simulink model "DualMotor_FaultTolerant_TorqueControl"  (R2025a)
settings: Solver=ode3  StartTime=0.0  StopTime=2  FixedStep=1e-6  RelTol=1e-3
libraries: spsDCVoltageSourceLib x2, spsGroundLib x2, eePmsmFieldOrientedControl x2, spsPermanentMagnetSynchronousMachineLib x2, spsUniversalBridgeLib x2, slpidlib x1, simulink x1, sps_lib x1
settings Model: Creator=lmh  LastModifiedBy=lmh

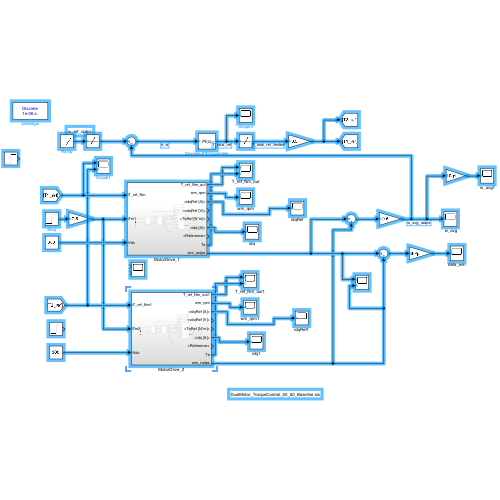
[thumbnail: Simulink's stored preview of the top-level diagram]
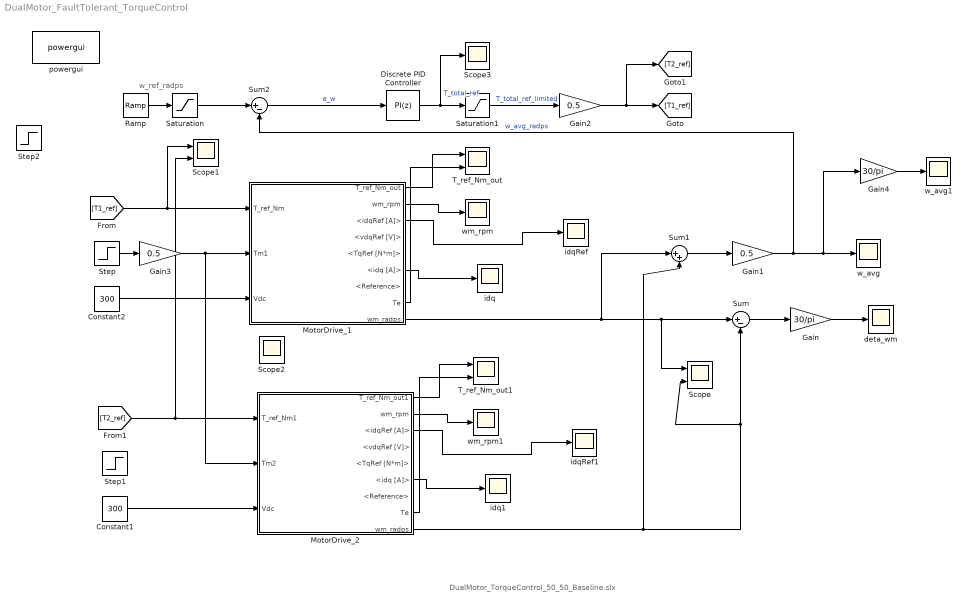
== system DualMotor_FaultTolerant_TorqueControl ==
  note: DualMotor_TorqueControl_50_50_Baseline.slx
  note: w_ref_radps
  " w_avg" : Scope
      settings: ActiveDisplayYMinimum=-1  ActiveDisplayYMaximum=1  DataLoggingVariableName=ScopeData10
  " w_avg1" : Scope
      settings: ActiveDisplayYMinimum=-42.23010556786226  ActiveDisplayYMaximum=380.07095011076035  DataLoggingVariableName=ScopeData11
  Constant1 : Constant  Value=300
  Constant2 : Constant  Value=300
  Discrete PID Controller : slpidlib/PID Controller  Controller=PI  Form=Parallel  TimeDomain=Discrete-time  UseExternalTs=off  SampleTime=1e-3  IntegratorMethod=Forward Euler  FilterMethod=Forward Euler  ControllerParametersSource=internal  P=0.2  I=0.3  UseKiTs=off  D=0  UseExternalDerivativeSource=off  N=100  UseFilter=on  TunerSelectOption=Transfer Function Based (PID Tuner App)  InitialConditionSource=internal  InitialConditionForIntegrator=0  InitialConditionForFilter=0  DifferentiatorICPrevScaledInput=0  ExternalReset=none  TrackingMode=off  Kt=1  LimitOutput=off  SatLimitsSource=internal  UpperSaturationLimit=inf  LowerSaturationLimit=-inf  LinearizeAsGain=off  AntiWindupMode=none  Kb=1  LimitIntegrator=off  UpperIntegratorSaturationLimit=inf  LowerIntegratorSaturationLimit=-inf  POutMin=[]  POutMax=[]  IOutMin=[]  IOutMax=[]  DOutMin=[]  DOutMax=[]  NOutMin=[]  NOutMax=[]  SumOutMin=[]  SumOutMax=[]  SaturationOutMin=[]  SaturationOutMax=[]  PParamMin=[]  PParamMax=[]  IParamMin=[]  IParamMax=[]  DParamMin=[]  DParamMax=[]  NParamMin=[]  NParamMax=[]  KbParamMin=[]  KbParamMax=[]  KtParamMin=[]  KtParamMax=[]  KbOutMin=[]  KbOutMax=[]  KtOutMin=[]  KtOutMax=[]  IntegratorOutMin=[]  IntegratorOutMax=[]  FilterOutMin=[]  FilterOutMax=[]  SumI1OutMin=[]  SumI1OutMax=[]  SumI2OutMin=[]  SumI2OutMax=[]  SumI3OutMin=[]  SumI3OutMax=[]  SumI4OutMin=[]  SumI4OutMax=[]  SumDOutMin=[]  SumDOutMax=[]  DifferentiatorOutMin=[]  DifferentiatorOutMax=[]  FilterDiffOutCoefMin=[]  FilterDiffOutCoefMax=[]  ReciprocalOutMin=[]  ReciprocalOutMax=[]  SumDenOutMin=[]  SumDenOutMax=[]  SumNumOutMin=[]  SumNumOutMax=[]  DivideOutMin=[]  DivideOutMax=[]  UdiffTsProdOutMin=[]  UdiffTsProdOutMax=[]  NTsProdOutMin=[]  NTsProdOutMax=[]  UintegralTsProdOutMin=[]  UintegralTsProdOutMax=[]  UngainTsProdOutMin=[]  UngainTsProdOutMax=[]  ClampingZeroOutDataTypeStr=Inherit: Inherit via back propagation  ClampingZeroOutMin=[]  ClampingZeroOutMax=[]  FilterDenConstantOutDataTypeStr=Inherit: Inherit via back propagation  FilterDenConstantOutMin=[]  FilterDenConstantOutMax=[]  PCopyOutDataTypeStr=Inherit: Inherit via back propagation  PCopyOutMin=[]  PCopyOutMax=[]  NCopyOutDataTypeStr=Inherit: Inherit via back propagation  NCopyOutMin=[]  NCopyOutMax=[]  IntegratorContinuousStateAttributes=''  IntegratorStateMustResolveToSignalObject=off  IntegratorRTWStateStorageClass=Auto  FilterContinuousStateAttributes=''  FilterStateMustResolveToSignalObject=off  FilterRTWStateStorageClass=Auto  ParallelPVariant=InternalParameters  IdealPVariant=Disabled  IVariant=InternalParameters  DVariant=Disabled  IntegratorVariant=Discrete  SatVariant=Disabled  AWVariant=Passthrough  PCopyVariant=Disabled  TRVariant=Disabled  FdbkBlocksVariant=Forward  IdealPFdbkVariant=Disabled  SatFdbkVariant=Disabled  DerivativeFilterVariant=Disabled  NVariant=Disabled  NCopyVariant=Disabled_SignalSpec  FilterICVariant=Disabled  IntegratorICVariant=InternalICs  ExternalResetVariant=Disabled  TRSumVariant=Passthrough  SumFdbkVariant=Disabled  SumVariant=Sum_PI  TsampFilterVariant=InternalTs  TsampNgainVariant=Passthrough  TsampIntegralVariant=Disabled_SignalSpec  ExternalSaturationOutDataTypeStr=Inherit: Same as second input  DerivativeSourceVariant=Disabled  PreIntVariant=InternalPreInt
      settings: LibrarySourceBlock=simulink/Discrete/Discrete PID Controller
  Gain : Gain  Gain=30/pi
  Gain1 : Gain  Gain=0.5
  Gain2 : Gain  Gain=0.5
  Gain3 : Gain  Gain=0.5
  Gain4 : Gain  Gain=30/pi
  MotorDrive_1 : Subsystem
  MotorDrive_2 : Subsystem
  Ramp : simulink/Sources/Ramp  slope=157.08  start=0.05  InitialOutput=0
  Saturation : Saturate  UpperLimit=31.416  LowerLimit=0
  Saturation1 : Saturate  UpperLimit=5  LowerLimit=-5
  Scope : Scope  NumInputPorts=2
      settings: ActiveDisplayYMinimum=-1  ActiveDisplayYMaximum=1  DataLoggingVariableName=ScopeData8
  Scope1 : Scope  NumInputPorts=2
      settings: ActiveDisplayYMinimum=-0.50042285131163777  ActiveDisplayYMaximum=0.992672654307302  DataLoggingVariableName=ScopeData12
  Scope2 : Scope  NumInputPorts=2
      settings: ActiveDisplayYMinimum=-0.40590531924916307  ActiveDisplayYMaximum=0.73013794484412364  DataLoggingVariableName=ScopeData13
  Scope3 : Scope
      settings: ActiveDisplayYMinimum=-0.97217317064289754  ActiveDisplayYMaximum=1.8423869448952914  DataLoggingVariableName=ScopeData14
  Step : Step  Time=0.3  SampleTime=1e-6
  Step1 : Step  Time=0.2  After=0.5  SampleTime=1e-6
  Step2 : Step  Time=0.2  After=0.5  SampleTime=1e-6
  Sum : Sum  Inputs=|+-
  Sum1 : Sum  Inputs=|++
  Sum2 : Sum  Inputs=|+-
  T_ref_Nm_out : Scope  NumInputPorts=2
      settings: ActiveDisplayYMinimum=-0.56957171237379067  ActiveDisplayYMaximum=1.0003558610919856
  T_ref_Nm_out1 : Scope  NumInputPorts=2
      settings: ActiveDisplayYMinimum=-1  ActiveDisplayYMaximum=1  DataLoggingVariableName=ScopeData6
  deta_wm : Scope
      settings: ActiveDisplayYMinimum=-1  ActiveDisplayYMaximum=1  DataLoggingVariableName=ScopeData9
  idq : Scope
      settings: ActiveDisplayYMinimum=-1.0831890867819363  ActiveDisplayYMaximum=1.2350252871725016  DataLoggingVariableName=ScopeData3
  idq1 : Scope
      settings: ActiveDisplayYMinimum=-0.803012654998282  ActiveDisplayYMaximum=1.1347435588564942  DataLoggingVariableName=ScopeData4
  idqRef : Scope
      settings: ActiveDisplayYMinimum=-0.26041666666666663  ActiveDisplayYMaximum=2.34375  DataLoggingVariableName=ScopeData2
  idqRef1 : Scope
      settings: ActiveDisplayYMinimum=-3.1835545787556114  ActiveDisplayYMaximum=2.3621352619007454  DataLoggingVariableName=ScopeData5
  powergui : sps_lib/powergui  Priority=1  SimulationMode=Discrete  SampleTime=1e-6  frequency=60  Iterations=50  frequencyindice=0  Pbase=100e6  ErrMax=1e-4  UnitsV=kV  UnitsW=MW  buscounter=0  FunctionMessages=off  echomessages=off  EnableUseOfTLC=off  CurrentSourceSwitches=off  DisableSnubberDevices=off  DisableRonSwitches=off  DisableVfSwitches=off  DisplayEquations=off  AutomaticDiscreteSolvers=off  SolverType=Tustin/Backward Euler (TBE)  Interpol=off  ExternalGateDelay=off  methode=off  Ts=100  x0status=blocks  SPID=on  SwTol=0  HookPort=off  NonlinearTolerance=1e-4  nMaxIteration=100  ContinueOnMaxIteration=off  RestoreLinks=warning  ResistiveCurrentMeasurement=off  Frange=[0:2:500]  Ylog=off  Xlog=on  ShowGrid=off  save=off  variable=ZData  structure=0  ZoomFFT=off  StartTime=0.0  cycles=1  DisplayStyle=1  fundamental=60  FreqAxis=off  MaxFrequency=1000  frequencyindicesteady=1  RmsSteady=1  display=off
  wm_rpm : Scope
      settings: ActiveDisplayYMinimum=-388.34435285098448  ActiveDisplayYMaximum=3465.7589265847746
  wm_rpm1 : Scope
      settings: ActiveDisplayYMinimum=-604.84980727002824  ActiveDisplayYMaximum=1187.9663788618518  DataLoggingVariableName=ScopeData7
  wires:
  Ramp/1 -> Saturation/1
  Sum/1 -> Gain/1
  MotorDrive_1/9(wm_radps) -> Sum1/1, Scope/1, Sum/1
  MotorDrive_2/3(<idqRef [A]>) -> idqRef1/1
  Step/1 -> Gain3/1
  MotorDrive_2/9(wm_radps) -> Scope/2, Sum/2, Sum1/2
  MotorDrive_2/1(T_ref_Nm_out1) -> T_ref_Nm_out1/1
  MotorDrive_2/2(wm_rpm) -> wm_rpm1/1
  Gain/1 -> deta_wm/1
  Constant2/1 -> MotorDrive_1/3(Vdc)
  MotorDrive_1/2(wm_rpm) -> wm_rpm/1
  Constant1/1 -> MotorDrive_2/3(Vdc)
  MotorDrive_1/1(T_ref_Nm_out) -> T_ref_Nm_out/1
  MotorDrive_1/6(<idq [A]>) -> idq/1
  MotorDrive_1/3(<idqRef [A]>) -> idqRef/1
  MotorDrive_2/6(<idq [A]>) -> idq1/1
  MotorDrive_1/8(Te) -> T_ref_Nm_out/2
  MotorDrive_2/8(Te) -> T_ref_Nm_out1/2
  Sum1/1 -> Gain1/1
  Gain1/1 -> Gain4/1, " w_avg"/1, Sum2/2  "w_avg_radps"
  Saturation/1 -> Sum2/1
  Sum2/1 -> Discrete PID Controller/1  "e_w"
  Discrete PID Controller/1 -> Scope3/1, Saturation1/1  "T_total_ref"
  Saturation1/1 -> Gain2/1  "T_total_ref_limited"
  Gain2/1 -> [T2_ref], [T1_ref]
  [T1_ref] -> Scope1/1, MotorDrive_1/1(T_ref_Nm)
  [T2_ref] -> Scope1/2, MotorDrive_2/1(T_ref_Nm1)
  Gain4/1 -> " w_avg1"/1
  Gain3/1 -> MotorDrive_2/2(Tm2), MotorDrive_1/2(Tm1)

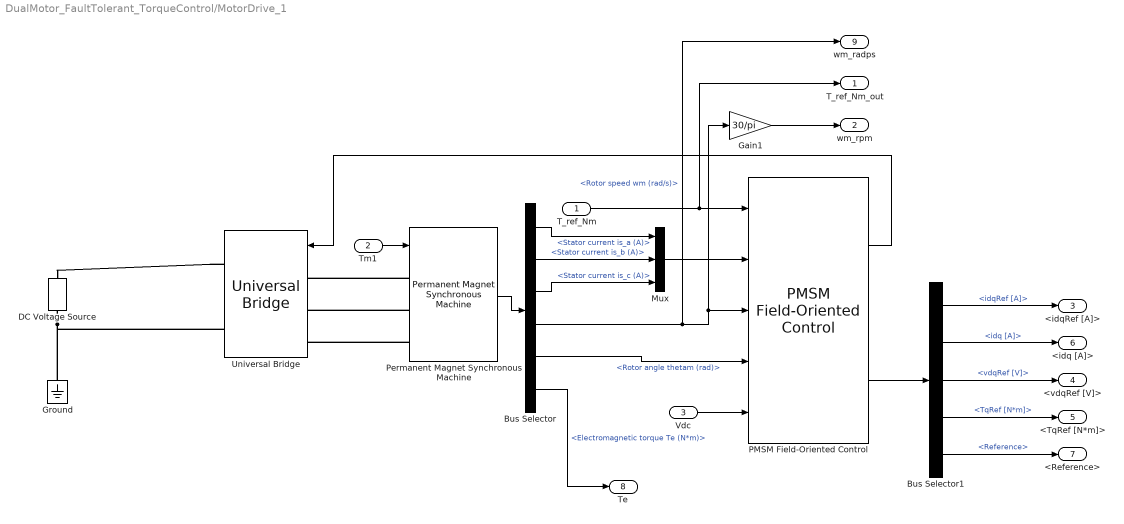
== system DualMotor_FaultTolerant_TorqueControl/MotorDrive_1 ==
  T_ref_Nm : Inport
  Tm1 : Inport  Port=2
  Vdc : Inport  Port=3
  Bus Selector : BusSelector  OutputSignals=Stator current is_a (A),Stator current is_b (A),Stator current is_c (A),Rotor speed wm (rad/s),Rotor angle thetam (rad),Electromagnetic torque Te (N*m)
  Bus Selector1 : BusSelector  OutputSignals=idqRef [A],idq [A],vdqRef [V],TqRef [N*m],Reference
  DC Voltage Source : spsDCVoltageSourceLib/DC Voltage Source  Amplitude=300  Measurements=None
  Gain1 : Gain  Gain=30/pi
  Ground : spsGroundLib/Ground  LConnTagsString=a
  Mux : Mux  Inputs=3
  PMSM Field-Oriented Control : eePmsmFieldOrientedControl/PMSM Field-Oriented Control  winding_type=Wye-wound  CtrlMode=Torque control  Vnom=300  Pmax=1000  Tmax=5  p=4  Vdc_on=50  Ts=1e-6  Tsc=1e-4  CtrlType=PI control  Kp_w=0.05  Ki_w=1  Kv_w=1  Kaw_w=1  RefType=Zero d-axis control  rpmVec=[0, 3000]  TqVec=[-100, 0, 100]  VdcVec=[300, 350]  PWMMode=SVM: space vector modulation  ModFactor=1  idMatrix=zeros(2,3,2)  iqMatrix=zeros(2,3,2)  psim=0.1194  Ld=0.00024  Lq=0.00029  Rs=0.01  AxisAlignment=Q-axis  Kp_id=4  Ki_id=30  Kaw_id=1  Kp_iq=4  Ki_iq=30  Kaw_iq=1  AxisPrio=Q-axis  ActZC=off  ActFF=on  ParamTypeFF=Constant parameters  LdFF=8.5e-3  LqFF=8.5e-3  psimFF=0.1194  idVect=[-200, 0, 200]  iqVect=[-200, 0, 200]  LdMatrix=0.0002 * ones(3, 3)  LqMatrix=0.0002 * ones(3, 3)  psimMatrix=0.04 * ones(3, 3)  CPWMMode=SVM: space vector modulation  fsw=10000
      settings: LibrarySourceBlock=|
      | ee_sl_lib/PMSM Control/PMSM Field-Oriented
      | Control
  Permanent Magnet Synchronous Machine : spsPermanentMagnetSynchronousMachineLib/Permanent Magnet Synchronous Machine  NbPhases=3  FluxDistribution=Sinusoidal  RotorType=Round  MechanicalLoad=Torque Tm  PresetModel=No  ShowDetailedParameters=on  MeasurementBus=off  Resistance=0.0485  Inductance=8.5e-3  dqInductances=[8.5e-3,8.5e-3]  La=8.5e-3  MachineConstant=Flux linkage established by magnets (V.s)  Flux=0.1194  VoltageCst=86.6271  TorqueCst=0.7164  Flat=120  Mechanical=[1e-3 1e-4 4 0]  PolePairs=4  InitialConditions=[0,0, 0,0]  InitialConditions5ph=[0 0 0 0 0 0]  RefAngle=90 degrees behind phase A axis (modified Park)  IterativeDiscreteModel=Trapezoidal non iterative  TsBlock=-1  TsPowergui=0
  Universal Bridge : spsUniversalBridgeLib/Universal Bridge  Arms=3  SnubberResistance=1e5  SnubberCapacitance=inf  Device=IGBT / Diodes  Ron=1e-3  Lon=0  ForwardVoltages="[  0  0  ]"  ForwardVoltage=0  GTOparameters=[ 10e-6 , 20e-6 ]  IGBTparameters=[ 1e-6 , 2e-6 ]  Measurements=None  Measurements_2=None  converterType=Rectifier
  T_ref_Nm_out : Outport
  wm_rpm : Outport  Port=2
  <idqRef [A]> : Outport  Port=3
  <vdqRef [V]> : Outport  Port=4
  <TqRef [N*m]> : Outport  Port=5
  <idq [A]> : Outport  Port=6
  <Reference> : Outport  Port=7
  Te : Outport  Port=8
  wm_radps : Outport  Port=9
  wires:
  Bus Selector1/4 -> <TqRef [N*m]>/1  "<TqRef [N*m]>"
  Permanent Magnet Synchronous Machine/1 -> Bus Selector/1
  Bus Selector/4 -> wm_radps/1, PMSM Field-Oriented Control/3, Gain1/1  "<Rotor speed wm (rad/s)>"
  Bus Selector/1 -> Mux/1  "<Stator current is_a (A)>"
  Bus Selector/3 -> Mux/3  "<Stator current is_c (A)>"
  PMSM Field-Oriented Control/2 -> Bus Selector1/1
  Mux/1 -> PMSM Field-Oriented Control/2
  Bus Selector/5 -> PMSM Field-Oriented Control/4  "<Rotor angle thetam (rad)>"
  Bus Selector/2 -> Mux/2  "<Stator current is_b (A)>"
  PMSM Field-Oriented Control/1 -> Universal Bridge/1
  Bus Selector1/2 -> <idq [A]>/1  "<idq [A]>"
  Bus Selector1/3 -> <vdqRef [V]>/1  "<vdqRef [V]>"
  Tm1/1 -> Permanent Magnet Synchronous Machine/1
  Bus Selector1/5 -> <Reference>/1  "<Reference>"
  Bus Selector1/1 -> <idqRef [A]>/1  "<idqRef [A]>"
  T_ref_Nm/1 -> T_ref_Nm_out/1, PMSM Field-Oriented Control/1
  Gain1/1 -> wm_rpm/1
  Vdc/1 -> PMSM Field-Oriented Control/5
  Bus Selector/6 -> Te/1  "<Electromagnetic torque Te (N*m)>"
  connections:
  Permanent Magnet Synchronous Machine/LConn3 -- Universal Bridge/LConn3
  DC Voltage Source/LConn1 -- Universal Bridge/RConn2 -- Ground/LConn1
  Permanent Magnet Synchronous Machine/LConn1 -- Universal Bridge/LConn1
  Permanent Magnet Synchronous Machine/LConn2 -- Universal Bridge/LConn2
  Universal Bridge/RConn1 -- DC Voltage Source/RConn1

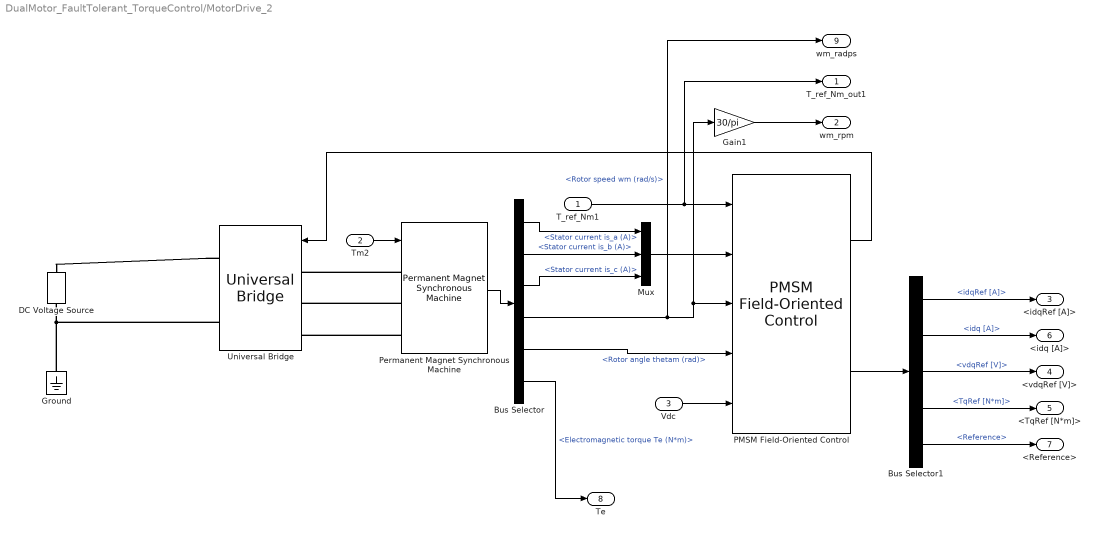
== system DualMotor_FaultTolerant_TorqueControl/MotorDrive_2 ==
  T_ref_Nm1 : Inport
  Tm2 : Inport  Port=2
  Vdc : Inport  Port=3
  Bus Selector : BusSelector  OutputSignals=Stator current is_a (A),Stator current is_b (A),Stator current is_c (A),Rotor speed wm (rad/s),Rotor angle thetam (rad),Electromagnetic torque Te (N*m)
  Bus Selector1 : BusSelector  OutputSignals=idqRef [A],idq [A],vdqRef [V],TqRef [N*m],Reference
  DC Voltage Source : spsDCVoltageSourceLib/DC Voltage Source  Amplitude=300  Measurements=None
  Gain1 : Gain  Gain=30/pi
  Ground : spsGroundLib/Ground  LConnTagsString=a
  Mux : Mux  Inputs=3
  PMSM Field-Oriented Control : eePmsmFieldOrientedControl/PMSM Field-Oriented Control  winding_type=Wye-wound  CtrlMode=Torque control  Vnom=300  Pmax=1000  Tmax=5  p=4  Vdc_on=50  Ts=1e-6  Tsc=1e-4  CtrlType=PI control  Kp_w=0.05  Ki_w=1  Kv_w=1  Kaw_w=1  RefType=Zero d-axis control  rpmVec=[0, 3000]  TqVec=[-100, 0, 100]  VdcVec=[300, 350]  PWMMode=SVM: space vector modulation  ModFactor=1  idMatrix=zeros(2,3,2)  iqMatrix=zeros(2,3,2)  psim=0.1194  Ld=0.00024  Lq=0.00029  Rs=0.01  AxisAlignment=Q-axis  Kp_id=4  Ki_id=30  Kaw_id=1  Kp_iq=4  Ki_iq=30  Kaw_iq=1  AxisPrio=Q-axis  ActZC=off  ActFF=on  ParamTypeFF=Constant parameters  LdFF=8.5e-3  LqFF=8.5e-3  psimFF=0.1194  idVect=[-200, 0, 200]  iqVect=[-200, 0, 200]  LdMatrix=0.0002 * ones(3, 3)  LqMatrix=0.0002 * ones(3, 3)  psimMatrix=0.04 * ones(3, 3)  CPWMMode=SVM: space vector modulation  fsw=10000
      settings: LibrarySourceBlock=|
      | ee_sl_lib/PMSM Control/PMSM Field-Oriented
      | Control
  Permanent Magnet Synchronous Machine : spsPermanentMagnetSynchronousMachineLib/Permanent Magnet Synchronous Machine  NbPhases=3  FluxDistribution=Sinusoidal  RotorType=Round  MechanicalLoad=Torque Tm  PresetModel=No  ShowDetailedParameters=on  MeasurementBus=off  Resistance=0.0485  Inductance=8.5e-3  dqInductances=[8.5e-3,8.5e-3]  La=8.5e-3  MachineConstant=Flux linkage established by magnets (V.s)  Flux=0.1194  VoltageCst=86.6271  TorqueCst=0.7164  Flat=120  Mechanical=[1e-3 1e-4 4 0]  PolePairs=4  InitialConditions=[0,0, 0,0]  InitialConditions5ph=[0 0 0 0 0 0]  RefAngle=90 degrees behind phase A axis (modified Park)  IterativeDiscreteModel=Trapezoidal non iterative  TsBlock=-1  TsPowergui=0
  Universal Bridge : spsUniversalBridgeLib/Universal Bridge  Arms=3  SnubberResistance=1e5  SnubberCapacitance=inf  Device=IGBT / Diodes  Ron=1e-3  Lon=0  ForwardVoltages="[  0  0  ]"  ForwardVoltage=0  GTOparameters=[ 10e-6 , 20e-6 ]  IGBTparameters=[ 1e-6 , 2e-6 ]  Measurements=None  Measurements_2=None  converterType=Rectifier
  T_ref_Nm_out1 : Outport
  wm_rpm : Outport  Port=2
  <idqRef [A]> : Outport  Port=3
  <vdqRef [V]> : Outport  Port=4
  <TqRef [N*m]> : Outport  Port=5
  <idq [A]> : Outport  Port=6
  <Reference> : Outport  Port=7
  Te : Outport  Port=8
  wm_radps : Outport  Port=9
  wires:
  Bus Selector/6 -> Te/1  "<Electromagnetic torque Te (N*m)>"
  Vdc/1 -> PMSM Field-Oriented Control/5
  Gain1/1 -> wm_rpm/1
  T_ref_Nm1/1 -> T_ref_Nm_out1/1, PMSM Field-Oriented Control/1
  Bus Selector1/1 -> <idqRef [A]>/1  "<idqRef [A]>"
  Bus Selector1/5 -> <Reference>/1  "<Reference>"
  Tm2/1 -> Permanent Magnet Synchronous Machine/1
  Bus Selector1/3 -> <vdqRef [V]>/1  "<vdqRef [V]>"
  Bus Selector1/2 -> <idq [A]>/1  "<idq [A]>"
  PMSM Field-Oriented Control/1 -> Universal Bridge/1
  Bus Selector/2 -> Mux/2  "<Stator current is_b (A)>"
  Bus Selector/5 -> PMSM Field-Oriented Control/4  "<Rotor angle thetam (rad)>"
  Mux/1 -> PMSM Field-Oriented Control/2
  PMSM Field-Oriented Control/2 -> Bus Selector1/1
  Bus Selector/3 -> Mux/3  "<Stator current is_c (A)>"
  Bus Selector/1 -> Mux/1  "<Stator current is_a (A)>"
  Bus Selector/4 -> Gain1/1, PMSM Field-Oriented Control/3, wm_radps/1  "<Rotor speed wm (rad/s)>"
  Permanent Magnet Synchronous Machine/1 -> Bus Selector/1
  Bus Selector1/4 -> <TqRef [N*m]>/1  "<TqRef [N*m]>"
  connections:
  Universal Bridge/RConn1 -- DC Voltage Source/RConn1
  Permanent Magnet Synchronous Machine/LConn2 -- Universal Bridge/LConn2
  Permanent Magnet Synchronous Machine/LConn1 -- Universal Bridge/LConn1
  Universal Bridge/RConn2 -- DC Voltage Source/LConn1 -- Ground/LConn1
  Permanent Magnet Synchronous Machine/LConn3 -- Universal Bridge/LConn3
